simulink model "double_pendulum1"  (Simulink 6.1)
settings: Solver=ode45  StartTime=0.0  StopTime=10.0  RelTol=1e-3
libraries: fuzblock x1
settings Model: LastModifiedBy=Administrator
settings DataIOCC: SignalLoggingName=sigsOut
settings OptimizationCC: BooleanDataType=off
settings HardwareCC: TargetUnknown=on

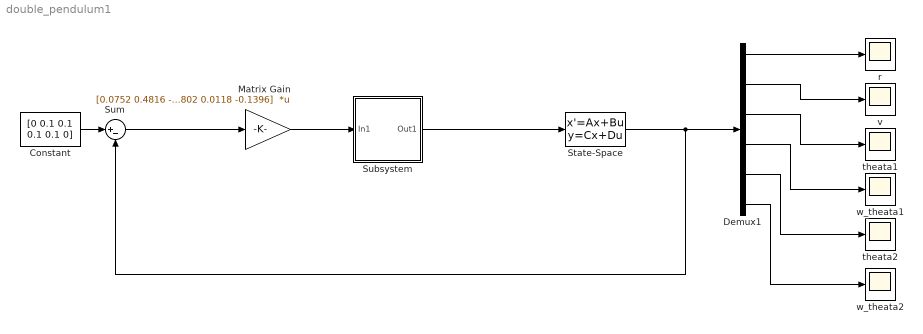
== system double_pendulum1 ==
  Constant : Constant  Value=[0 0.1 0.1 0.1 0.1 0]
  Demux1 : Demux  Outputs=6
  Matrix Gain : Gain  Gain=[0.0752 0.4816 -0.8581 0 0 0;0 0 0 0.0802 0.0118 -0.1396]  Multiplication=Matrix(K*u)  SaturateOnIntegerOverflow=on
  State-Space : StateSpace  A=[0 0 0 1 0 0;0 0 0 0 1 0;0 0 0 0 0 1;0 0 0 0 0 0;0 86.69 -21.62 0 0 0;0 -40.31 39.45 0 0 0]  B=[0 0 0 1 6.64 -0.088]'  C=[1 0 0 0 0 0;0 1 0 0 0 0;0 0 1 0 0 0;0 0 0 1 0 0;0 0 0 0 1 0;0 0 0 0 0 1]  D=[0 0 0 0 0 0]'
  Subsystem : Subsystem  mask{Ke=10, Kec=10, Ku=24}
      mask Display: disp('fuzzy\nController')
  Sum : Sum  Inputs=|+-  SaturateOnIntegerOverflow=on
  r : Scope
      settings: TimeRange=10  YMin=-0.8  YMax=0.15
  theata1 : Scope
      settings: TimeRange=10  YMin=-0.8  YMax=0.15  SaveName=ScopeData2
  theata2 : Scope
      settings: TimeRange=10  YMin=-0.8  YMax=0.15  SaveName=ScopeData4
  v : Scope
      settings: TimeRange=10  YMin=-0.8  YMax=0.15
  w_theata1 : Scope
      settings: TimeRange=10  YMin=-0.8  YMax=0.15  SaveName=ScopeData3
  w_theata2 : Scope
      settings: TimeRange=10  YMin=-0.8  YMax=0.15  SaveName=ScopeData5
  wires:
  Constant/1 -> Sum/1
  Demux1/1 -> r/1
  Matrix Gain/1 -> Subsystem/1(In1)
  Demux1/2 -> v/1
  Demux1/3 -> theata1/1
  Demux1/4 -> w_theata1/1
  Demux1/5 -> theata2/1
  Demux1/6 -> w_theata2/1
  State-Space/1 -> Sum/2, Demux1/1
  Subsystem/1(Out1) -> State-Space/1
  Sum/1 -> Matrix Gain/1

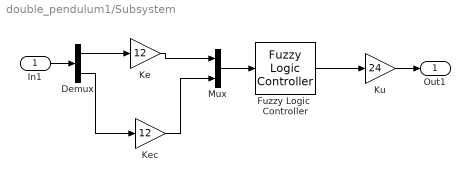
== system double_pendulum1/Subsystem ==
  In1 : Inport  Port=1  LatchInput=off
  Demux : Demux  Outputs=2
  Fuzzy Logic  Controller : fuzblock/Fuzzy Logic  Controller  fis=fismat
  Ke : Gain  Gain=12  SaturateOnIntegerOverflow=on
  Kec : Gain  Gain=12  SaturateOnIntegerOverflow=on
  Ku : Gain  Gain=24  SaturateOnIntegerOverflow=on
  Mux : Mux  Inputs=2
  Out1 : Outport
  wires:
  Ke/1 -> Mux/1
  Kec/1 -> Mux/2
  Mux/1 -> Fuzzy Logic  Controller/1
  Fuzzy Logic  Controller/1 -> Ku/1
  Demux/1 -> Ke/1
  Demux/2 -> Kec/1
  In1/1 -> Demux/1
  Ku/1 -> Out1/1
